simulink model "cic_filter_testing_8"  (Simulink 7.4)
settings: Solver=ode45  StartTime=0.0  StopTime=10000  RelTol=1e-3
undefined symbols (not defined in the file or in its folder): xlRetrieveParam
libraries: xbsIndex_r4 x441
(part 2 of 3)

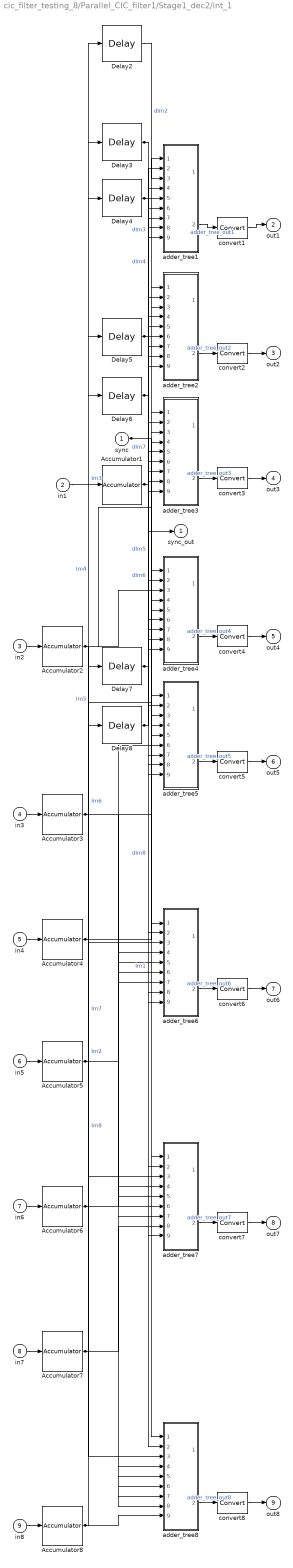
== system cic_filter_testing_8/Parallel_CIC_filter1/Stage1_dec2/int_1 ==
  sync : Inport
  in1 : Inport  Port=2
  in2 : Inport  Port=3
  in3 : Inport  Port=4
  in4 : Inport  Port=5
  in5 : Inport  Port=6
  in6 : Inport  Port=7
  in7 : Inport  Port=8
  in8 : Inport  Port=9
  Accumulator{1..8} (8 alike) : xbsIndex_r4/Accumulator  operation=Add  n_bits=11  overflow=Wrap  scale=1  rst=off  hasbypass=off  en=off  dbl_ovrd=off  use_behavioral_HDL=on  implementation=Fabric  block_type=accum
      settings: block_version=11.4
  Delay{2..8} (7 alike) : xbsIndex_r4/Delay  en=off  latency=1  dbl_ovrd=off  reg_retiming=off  block_type=delay
      settings: block_version=11.4
  adder_tree1 : Subsystem
  adder_tree2 : Subsystem
  adder_tree3 : Subsystem
  adder_tree4 : Subsystem
  adder_tree5 : Subsystem
  adder_tree6 : Subsystem
  adder_tree7 : Subsystem
  adder_tree8 : Subsystem
  convert{1..8} (8 alike) : xbsIndex_r4/Convert  arith_type="Signed  (2's comp)"  n_bits=11  bin_pt=7  quantization=Truncate  overflow=Wrap  latency=0  dbl_ovrd=off  pipeline=off  block_type=convert
      settings: block_version=11.4
  sync_out : Outport
  out1 : Outport  Port=2
  out2 : Outport  Port=3
  out3 : Outport  Port=4
  out4 : Outport  Port=5
  out5 : Outport  Port=6
  out6 : Outport  Port=7
  out7 : Outport  Port=8
  out8 : Outport  Port=9
  wires:
  Accumulator2/1 -> adder_tree8/3(din_2), adder_tree7/3(din_2), adder_tree6/3(din_2), adder_tree5/3(din_2), adder_tree4/3(din_2), adder_tree3/3(din_2), adder_tree2/3(din_2), Delay2/1  "Im2"
  Accumulator3/1 -> adder_tree8/4(din_3), adder_tree7/4(din_3), adder_tree6/4(din_3), adder_tree5/4(din_3), adder_tree4/4(din_3), adder_tree3/4(din_3), Delay3/1  "Im3"
  Accumulator4/1 -> adder_tree8/5(din_4), adder_tree7/5(din_4), adder_tree6/5(din_4), adder_tree5/5(din_4), adder_tree4/5(din_4), Delay4/1  "Im4"
  Accumulator5/1 -> adder_tree8/6(din_5), adder_tree7/6(din_5), adder_tree6/6(din_5), adder_tree5/6(din_5), Delay5/1  "Im5"
  Accumulator6/1 -> adder_tree8/7(din_6), adder_tree7/7(din_6), adder_tree6/7(din_6), Delay6/1  "Im6"
  Accumulator7/1 -> adder_tree8/8(din_7), adder_tree7/8(din_7), Delay7/1  "Im7"
  Accumulator8/1 -> adder_tree8/9(din_8), Delay8/1  "Im8"
  sync/1 -> sync_out/1, adder_tree8/1(sync), adder_tree7/1(sync), adder_tree6/1(sync), adder_tree5/1(sync), adder_tree4/1(sync), adder_tree3/1(sync), adder_tree2/1(sync), adder_tree1/1(sync)
  Accumulator1/1 -> adder_tree8/2(din_1), adder_tree7/2(din_1), adder_tree6/2(din_1), adder_tree5/2(din_1), adder_tree4/2(din_1), adder_tree3/2(din_1), adder_tree2/2(din_1), adder_tree1/2(din_1)  "Im1"
  Delay3/1 -> adder_tree2/4(din_3), adder_tree1/4(din_3)  "dIm3"
  Delay4/1 -> adder_tree3/5(din_4), adder_tree2/5(din_4), adder_tree1/5(din_4)  "dIm4"
  Delay5/1 -> adder_tree4/6(din_5), adder_tree3/6(din_5), adder_tree2/6(din_5), adder_tree1/6(din_5)  "dIm5"
  Delay6/1 -> adder_tree5/7(din_6), adder_tree4/7(din_6), adder_tree3/7(din_6), adder_tree2/7(din_6), adder_tree1/7(din_6)  "dIm6"
  Delay7/1 -> adder_tree6/8(din_7), adder_tree5/8(din_7), adder_tree4/8(din_7), adder_tree3/8(din_7), adder_tree2/8(din_7), adder_tree1/8(din_7)  "dIm7"
  Delay8/1 -> adder_tree7/9(din_8), adder_tree6/9(din_8), adder_tree5/9(din_8), adder_tree4/9(din_8), adder_tree3/9(din_8), adder_tree2/9(din_8), adder_tree1/9(din_8)  "dIm8"
  convert8/1 -> out8/1
  adder_tree8/2(dout) -> convert8/1  "adder_tree_out8"
  convert7/1 -> out7/1
  adder_tree7/2(dout) -> convert7/1  "adder_tree_out7"
  convert6/1 -> out6/1
  adder_tree6/2(dout) -> convert6/1  "adder_tree_out6"
  convert5/1 -> out5/1
  adder_tree5/2(dout) -> convert5/1  "adder_tree_out5"
  convert4/1 -> out4/1
  adder_tree4/2(dout) -> convert4/1  "adder_tree_out4"
  convert3/1 -> out3/1
  adder_tree3/2(dout) -> convert3/1  "adder_tree_out3"
  convert2/1 -> out2/1
  adder_tree2/2(dout) -> convert2/1  "adder_tree_out2"
  convert1/1 -> out1/1
  adder_tree1/2(dout) -> convert1/1  "adder_tree_out1"
  Delay2/1 -> adder_tree1/3(din_2)  "dIm2"
  in8/1 -> Accumulator8/1
  in7/1 -> Accumulator7/1
  in6/1 -> Accumulator6/1
  in5/1 -> Accumulator5/1
  in4/1 -> Accumulator4/1
  in3/1 -> Accumulator3/1
  in2/1 -> Accumulator2/1
  in1/1 -> Accumulator1/1

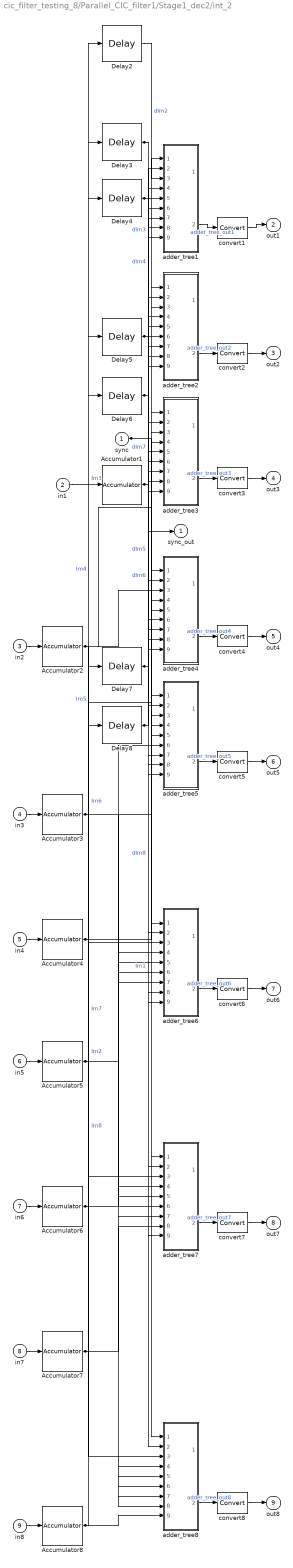
== system cic_filter_testing_8/Parallel_CIC_filter1/Stage1_dec2/int_2 ==
  sync : Inport
  in1 : Inport  Port=2
  in2 : Inport  Port=3
  in3 : Inport  Port=4
  in4 : Inport  Port=5
  in5 : Inport  Port=6
  in6 : Inport  Port=7
  in7 : Inport  Port=8
  in8 : Inport  Port=9
  Accumulator{1..8} (8 alike) : xbsIndex_r4/Accumulator  operation=Add  n_bits=11  overflow=Wrap  scale=1  rst=off  hasbypass=off  en=off  dbl_ovrd=off  use_behavioral_HDL=on  implementation=Fabric  block_type=accum
      settings: block_version=11.4
  Delay{2..8} (7 alike) : xbsIndex_r4/Delay  en=off  latency=1  dbl_ovrd=off  reg_retiming=off  block_type=delay
      settings: block_version=11.4
  adder_tree1 : Subsystem
  adder_tree2 : Subsystem
  adder_tree3 : Subsystem
  adder_tree4 : Subsystem
  adder_tree5 : Subsystem
  adder_tree6 : Subsystem
  adder_tree7 : Subsystem
  adder_tree8 : Subsystem
  convert{1..8} (8 alike) : xbsIndex_r4/Convert  arith_type="Signed  (2's comp)"  n_bits=11  bin_pt=7  quantization=Truncate  overflow=Wrap  latency=0  dbl_ovrd=off  pipeline=off  block_type=convert
      settings: block_version=11.4
  sync_out : Outport
  out1 : Outport  Port=2
  out2 : Outport  Port=3
  out3 : Outport  Port=4
  out4 : Outport  Port=5
  out5 : Outport  Port=6
  out6 : Outport  Port=7
  out7 : Outport  Port=8
  out8 : Outport  Port=9
  wires:
  Accumulator2/1 -> adder_tree8/3(din_2), adder_tree7/3(din_2), adder_tree6/3(din_2), adder_tree5/3(din_2), adder_tree4/3(din_2), adder_tree3/3(din_2), adder_tree2/3(din_2), Delay2/1  "Im2"
  Accumulator3/1 -> adder_tree8/4(din_3), adder_tree7/4(din_3), adder_tree6/4(din_3), adder_tree5/4(din_3), adder_tree4/4(din_3), adder_tree3/4(din_3), Delay3/1  "Im3"
  Accumulator4/1 -> adder_tree8/5(din_4), adder_tree7/5(din_4), adder_tree6/5(din_4), adder_tree5/5(din_4), adder_tree4/5(din_4), Delay4/1  "Im4"
  Accumulator5/1 -> adder_tree8/6(din_5), adder_tree7/6(din_5), adder_tree6/6(din_5), adder_tree5/6(din_5), Delay5/1  "Im5"
  Accumulator6/1 -> adder_tree8/7(din_6), adder_tree7/7(din_6), adder_tree6/7(din_6), Delay6/1  "Im6"
  Accumulator7/1 -> adder_tree8/8(din_7), adder_tree7/8(din_7), Delay7/1  "Im7"
  Accumulator8/1 -> adder_tree8/9(din_8), Delay8/1  "Im8"
  sync/1 -> sync_out/1, adder_tree8/1(sync), adder_tree7/1(sync), adder_tree6/1(sync), adder_tree5/1(sync), adder_tree4/1(sync), adder_tree3/1(sync), adder_tree2/1(sync), adder_tree1/1(sync)
  Accumulator1/1 -> adder_tree8/2(din_1), adder_tree7/2(din_1), adder_tree6/2(din_1), adder_tree5/2(din_1), adder_tree4/2(din_1), adder_tree3/2(din_1), adder_tree2/2(din_1), adder_tree1/2(din_1)  "Im1"
  Delay3/1 -> adder_tree2/4(din_3), adder_tree1/4(din_3)  "dIm3"
  Delay4/1 -> adder_tree3/5(din_4), adder_tree2/5(din_4), adder_tree1/5(din_4)  "dIm4"
  Delay5/1 -> adder_tree4/6(din_5), adder_tree3/6(din_5), adder_tree2/6(din_5), adder_tree1/6(din_5)  "dIm5"
  Delay6/1 -> adder_tree5/7(din_6), adder_tree4/7(din_6), adder_tree3/7(din_6), adder_tree2/7(din_6), adder_tree1/7(din_6)  "dIm6"
  Delay7/1 -> adder_tree6/8(din_7), adder_tree5/8(din_7), adder_tree4/8(din_7), adder_tree3/8(din_7), adder_tree2/8(din_7), adder_tree1/8(din_7)  "dIm7"
  Delay8/1 -> adder_tree7/9(din_8), adder_tree6/9(din_8), adder_tree5/9(din_8), adder_tree4/9(din_8), adder_tree3/9(din_8), adder_tree2/9(din_8), adder_tree1/9(din_8)  "dIm8"
  convert8/1 -> out8/1
  adder_tree8/2(dout) -> convert8/1  "adder_tree_out8"
  convert7/1 -> out7/1
  adder_tree7/2(dout) -> convert7/1  "adder_tree_out7"
  convert6/1 -> out6/1
  adder_tree6/2(dout) -> convert6/1  "adder_tree_out6"
  convert5/1 -> out5/1
  adder_tree5/2(dout) -> convert5/1  "adder_tree_out5"
  convert4/1 -> out4/1
  adder_tree4/2(dout) -> convert4/1  "adder_tree_out4"
  convert3/1 -> out3/1
  adder_tree3/2(dout) -> convert3/1  "adder_tree_out3"
  convert2/1 -> out2/1
  adder_tree2/2(dout) -> convert2/1  "adder_tree_out2"
  convert1/1 -> out1/1
  adder_tree1/2(dout) -> convert1/1  "adder_tree_out1"
  Delay2/1 -> adder_tree1/3(din_2)  "dIm2"
  in8/1 -> Accumulator8/1
  in7/1 -> Accumulator7/1
  in6/1 -> Accumulator6/1
  in5/1 -> Accumulator5/1
  in4/1 -> Accumulator4/1
  in3/1 -> Accumulator3/1
  in2/1 -> Accumulator2/1
  in1/1 -> Accumulator1/1

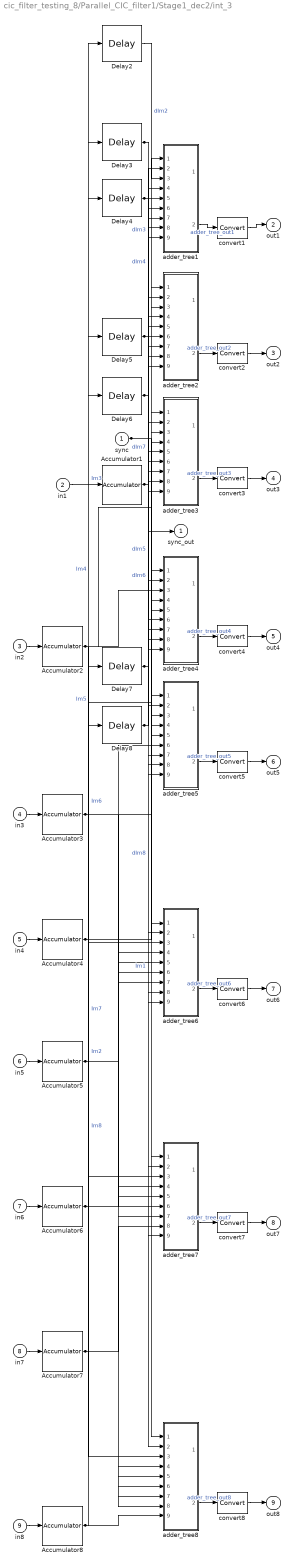
== system cic_filter_testing_8/Parallel_CIC_filter1/Stage1_dec2/int_3 ==
  sync : Inport
  in1 : Inport  Port=2
  in2 : Inport  Port=3
  in3 : Inport  Port=4
  in4 : Inport  Port=5
  in5 : Inport  Port=6
  in6 : Inport  Port=7
  in7 : Inport  Port=8
  in8 : Inport  Port=9
  Accumulator{1..8} (8 alike) : xbsIndex_r4/Accumulator  operation=Add  n_bits=11  overflow=Wrap  scale=1  rst=off  hasbypass=off  en=off  dbl_ovrd=off  use_behavioral_HDL=on  implementation=Fabric  block_type=accum
      settings: block_version=11.4
  Delay{2..8} (7 alike) : xbsIndex_r4/Delay  en=off  latency=1  dbl_ovrd=off  reg_retiming=off  block_type=delay
      settings: block_version=11.4
  adder_tree1 : Subsystem
  adder_tree2 : Subsystem
  adder_tree3 : Subsystem
  adder_tree4 : Subsystem
  adder_tree5 : Subsystem
  adder_tree6 : Subsystem
  adder_tree7 : Subsystem
  adder_tree8 : Subsystem
  convert{1..8} (8 alike) : xbsIndex_r4/Convert  arith_type="Signed  (2's comp)"  n_bits=11  bin_pt=7  quantization=Truncate  overflow=Wrap  latency=0  dbl_ovrd=off  pipeline=off  block_type=convert
      settings: block_version=11.4
  sync_out : Outport
  out1 : Outport  Port=2
  out2 : Outport  Port=3
  out3 : Outport  Port=4
  out4 : Outport  Port=5
  out5 : Outport  Port=6
  out6 : Outport  Port=7
  out7 : Outport  Port=8
  out8 : Outport  Port=9
  wires:
  Accumulator2/1 -> adder_tree8/3(din_2), adder_tree7/3(din_2), adder_tree6/3(din_2), adder_tree5/3(din_2), adder_tree4/3(din_2), adder_tree3/3(din_2), adder_tree2/3(din_2), Delay2/1  "Im2"
  Accumulator3/1 -> adder_tree8/4(din_3), adder_tree7/4(din_3), adder_tree6/4(din_3), adder_tree5/4(din_3), adder_tree4/4(din_3), adder_tree3/4(din_3), Delay3/1  "Im3"
  Accumulator4/1 -> adder_tree8/5(din_4), adder_tree7/5(din_4), adder_tree6/5(din_4), adder_tree5/5(din_4), adder_tree4/5(din_4), Delay4/1  "Im4"
  Accumulator5/1 -> adder_tree8/6(din_5), adder_tree7/6(din_5), adder_tree6/6(din_5), adder_tree5/6(din_5), Delay5/1  "Im5"
  Accumulator6/1 -> adder_tree8/7(din_6), adder_tree7/7(din_6), adder_tree6/7(din_6), Delay6/1  "Im6"
  Accumulator7/1 -> adder_tree8/8(din_7), adder_tree7/8(din_7), Delay7/1  "Im7"
  Accumulator8/1 -> adder_tree8/9(din_8), Delay8/1  "Im8"
  sync/1 -> sync_out/1, adder_tree8/1(sync), adder_tree7/1(sync), adder_tree6/1(sync), adder_tree5/1(sync), adder_tree4/1(sync), adder_tree3/1(sync), adder_tree2/1(sync), adder_tree1/1(sync)
  Accumulator1/1 -> adder_tree8/2(din_1), adder_tree7/2(din_1), adder_tree6/2(din_1), adder_tree5/2(din_1), adder_tree4/2(din_1), adder_tree3/2(din_1), adder_tree2/2(din_1), adder_tree1/2(din_1)  "Im1"
  Delay3/1 -> adder_tree2/4(din_3), adder_tree1/4(din_3)  "dIm3"
  Delay4/1 -> adder_tree3/5(din_4), adder_tree2/5(din_4), adder_tree1/5(din_4)  "dIm4"
  Delay5/1 -> adder_tree4/6(din_5), adder_tree3/6(din_5), adder_tree2/6(din_5), adder_tree1/6(din_5)  "dIm5"
  Delay6/1 -> adder_tree5/7(din_6), adder_tree4/7(din_6), adder_tree3/7(din_6), adder_tree2/7(din_6), adder_tree1/7(din_6)  "dIm6"
  Delay7/1 -> adder_tree6/8(din_7), adder_tree5/8(din_7), adder_tree4/8(din_7), adder_tree3/8(din_7), adder_tree2/8(din_7), adder_tree1/8(din_7)  "dIm7"
  Delay8/1 -> adder_tree7/9(din_8), adder_tree6/9(din_8), adder_tree5/9(din_8), adder_tree4/9(din_8), adder_tree3/9(din_8), adder_tree2/9(din_8), adder_tree1/9(din_8)  "dIm8"
  convert8/1 -> out8/1
  adder_tree8/2(dout) -> convert8/1  "adder_tree_out8"
  convert7/1 -> out7/1
  adder_tree7/2(dout) -> convert7/1  "adder_tree_out7"
  convert6/1 -> out6/1
  adder_tree6/2(dout) -> convert6/1  "adder_tree_out6"
  convert5/1 -> out5/1
  adder_tree5/2(dout) -> convert5/1  "adder_tree_out5"
  convert4/1 -> out4/1
  adder_tree4/2(dout) -> convert4/1  "adder_tree_out4"
  convert3/1 -> out3/1
  adder_tree3/2(dout) -> convert3/1  "adder_tree_out3"
  convert2/1 -> out2/1
  adder_tree2/2(dout) -> convert2/1  "adder_tree_out2"
  convert1/1 -> out1/1
  adder_tree1/2(dout) -> convert1/1  "adder_tree_out1"
  Delay2/1 -> adder_tree1/3(din_2)  "dIm2"
  in8/1 -> Accumulator8/1
  in7/1 -> Accumulator7/1
  in6/1 -> Accumulator6/1
  in5/1 -> Accumulator5/1
  in4/1 -> Accumulator4/1
  in3/1 -> Accumulator3/1
  in2/1 -> Accumulator2/1
  in1/1 -> Accumulator1/1

== system cic_filter_testing_8/Parallel_CIC_filter1/Stage2_dec2/comb_1 ==
  sync_in : Inport
  in1 : Inport  Port=2
  in2 : Inport  Port=3
  Delay2 : xbsIndex_r4/Delay  en=off  latency=1  dbl_ovrd=off  reg_retiming=off  block_type=delay
      settings: block_version=11.4
  sub_blk1 : xbsIndex_r4/AddSub  mode=Subtraction  use_carryin=off  use_carryout=off  en=off  latency=1  precision=User Defined  arith_type="Signed  (2's comp)"  n_bits=14  bin_pt=7  quantization=Truncate  overflow=Wrap  dbl_ovrd=off  use_behavioral_HDL=on  hw_selection=Fabric  pipelined=off  block_type=addsub
  sub_blk2 : xbsIndex_r4/AddSub  mode=Subtraction  use_carryin=off  use_carryout=off  en=off  latency=1  precision=User Defined  arith_type="Signed  (2's comp)"  n_bits=14  bin_pt=7  quantization=Truncate  overflow=Wrap  dbl_ovrd=off  use_behavioral_HDL=on  hw_selection=Fabric  pipelined=off  block_type=addsub
  sync_delay : xbsIndex_r4/Delay  en=off  latency=1  dbl_ovrd=off  reg_retiming=off  block_type=delay
      settings: block_version=11.4
  sync_out : Outport
  out1 : Outport  Port=2
  out2 : Outport  Port=3
  wires:
  in2/1 -> sub_blk2/1, Delay2/1
  in1/1 -> sub_blk2/2, sub_blk1/1
  sync_delay/1 -> sync_out/1
  sync_in/1 -> sync_delay/1
  sub_blk2/1 -> out2/1
  sub_blk1/1 -> out1/1
  Delay2/1 -> sub_blk1/2  "d_in2"

== system cic_filter_testing_8/Parallel_CIC_filter1/Stage2_dec2/comb_2 ==
  sync_in : Inport
  in1 : Inport  Port=2
  in2 : Inport  Port=3
  Delay2 : xbsIndex_r4/Delay  en=off  latency=1  dbl_ovrd=off  reg_retiming=off  block_type=delay
      settings: block_version=11.4
  sub_blk1 : xbsIndex_r4/AddSub  mode=Subtraction  use_carryin=off  use_carryout=off  en=off  latency=1  precision=User Defined  arith_type="Signed  (2's comp)"  n_bits=14  bin_pt=7  quantization=Truncate  overflow=Wrap  dbl_ovrd=off  use_behavioral_HDL=on  hw_selection=Fabric  pipelined=off  block_type=addsub
  sub_blk2 : xbsIndex_r4/AddSub  mode=Subtraction  use_carryin=off  use_carryout=off  en=off  latency=1  precision=User Defined  arith_type="Signed  (2's comp)"  n_bits=14  bin_pt=7  quantization=Truncate  overflow=Wrap  dbl_ovrd=off  use_behavioral_HDL=on  hw_selection=Fabric  pipelined=off  block_type=addsub
  sync_delay : xbsIndex_r4/Delay  en=off  latency=1  dbl_ovrd=off  reg_retiming=off  block_type=delay
      settings: block_version=11.4
  sync_out : Outport
  out1 : Outport  Port=2
  out2 : Outport  Port=3
  wires:
  in2/1 -> sub_blk2/1, Delay2/1
  in1/1 -> sub_blk2/2, sub_blk1/1
  sync_delay/1 -> sync_out/1
  sync_in/1 -> sync_delay/1
  sub_blk2/1 -> out2/1
  sub_blk1/1 -> out1/1
  Delay2/1 -> sub_blk1/2  "d_in2"

== system cic_filter_testing_8/Parallel_CIC_filter1/Stage2_dec2/comb_3 ==
  sync_in : Inport
  in1 : Inport  Port=2
  in2 : Inport  Port=3
  Delay2 : xbsIndex_r4/Delay  en=off  latency=1  dbl_ovrd=off  reg_retiming=off  block_type=delay
      settings: block_version=11.4
  sub_blk1 : xbsIndex_r4/AddSub  mode=Subtraction  use_carryin=off  use_carryout=off  en=off  latency=1  precision=User Defined  arith_type="Signed  (2's comp)"  n_bits=14  bin_pt=7  quantization=Truncate  overflow=Wrap  dbl_ovrd=off  use_behavioral_HDL=on  hw_selection=Fabric  pipelined=off  block_type=addsub
  sub_blk2 : xbsIndex_r4/AddSub  mode=Subtraction  use_carryin=off  use_carryout=off  en=off  latency=1  precision=User Defined  arith_type="Signed  (2's comp)"  n_bits=14  bin_pt=7  quantization=Truncate  overflow=Wrap  dbl_ovrd=off  use_behavioral_HDL=on  hw_selection=Fabric  pipelined=off  block_type=addsub
  sync_delay : xbsIndex_r4/Delay  en=off  latency=1  dbl_ovrd=off  reg_retiming=off  block_type=delay
      settings: block_version=11.4
  sync_out : Outport
  out1 : Outport  Port=2
  out2 : Outport  Port=3
  wires:
  in2/1 -> sub_blk2/1, Delay2/1
  in1/1 -> sub_blk2/2, sub_blk1/1
  sync_delay/1 -> sync_out/1
  sync_in/1 -> sync_delay/1
  sub_blk2/1 -> out2/1
  sub_blk1/1 -> out1/1
  Delay2/1 -> sub_blk1/2  "d_in2"

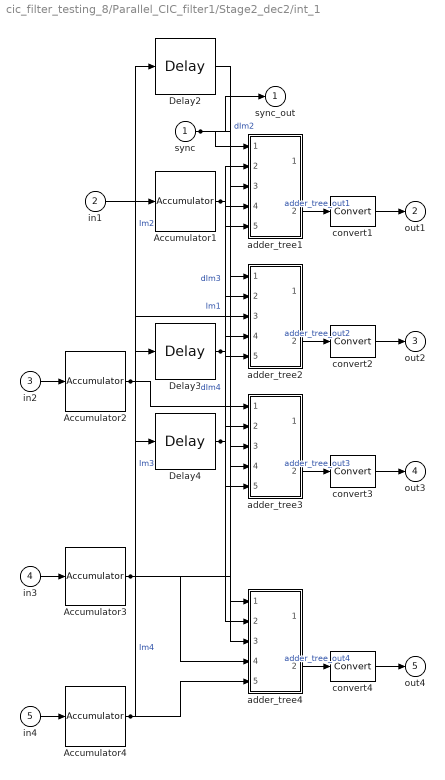
== system cic_filter_testing_8/Parallel_CIC_filter1/Stage2_dec2/int_1 ==
  sync : Inport
  in1 : Inport  Port=2
  in2 : Inport  Port=3
  in3 : Inport  Port=4
  in4 : Inport  Port=5
  Accumulator{1..4} (4 alike) : xbsIndex_r4/Accumulator  operation=Add  n_bits=14  overflow=Wrap  scale=1  rst=off  hasbypass=off  en=off  dbl_ovrd=off  use_behavioral_HDL=on  implementation=Fabric  block_type=accum
      settings: block_version=11.4
  Delay2 : xbsIndex_r4/Delay  en=off  latency=1  dbl_ovrd=off  reg_retiming=off  block_type=delay
      settings: block_version=11.4
  Delay3 : xbsIndex_r4/Delay  en=off  latency=1  dbl_ovrd=off  reg_retiming=off  block_type=delay
      settings: block_version=11.4
  Delay4 : xbsIndex_r4/Delay  en=off  latency=1  dbl_ovrd=off  reg_retiming=off  block_type=delay
      settings: block_version=11.4
  adder_tree1 : Subsystem
  adder_tree2 : Subsystem
  adder_tree3 : Subsystem
  adder_tree4 : Subsystem
  convert{1..4} (4 alike) : xbsIndex_r4/Convert  arith_type="Signed  (2's comp)"  n_bits=14  bin_pt=7  quantization=Truncate  overflow=Wrap  latency=0  dbl_ovrd=off  pipeline=off  block_type=convert
      settings: block_version=11.4
  sync_out : Outport
  out1 : Outport  Port=2
  out2 : Outport  Port=3
  out3 : Outport  Port=4
  out4 : Outport  Port=5
  wires:
  Accumulator2/1 -> adder_tree4/3(din_2), adder_tree3/3(din_2), adder_tree2/3(din_2), Delay2/1  "Im2"
  Accumulator3/1 -> adder_tree4/4(din_3), adder_tree3/4(din_3), Delay3/1  "Im3"
  Accumulator4/1 -> adder_tree4/5(din_4), Delay4/1  "Im4"
  sync/1 -> sync_out/1, adder_tree4/1(sync), adder_tree3/1(sync), adder_tree2/1(sync), adder_tree1/1(sync)
  Accumulator1/1 -> adder_tree4/2(din_1), adder_tree3/2(din_1), adder_tree2/2(din_1), adder_tree1/2(din_1)  "Im1"
  Delay3/1 -> adder_tree2/4(din_3), adder_tree1/4(din_3)  "dIm3"
  Delay4/1 -> adder_tree3/5(din_4), adder_tree2/5(din_4), adder_tree1/5(din_4)  "dIm4"
  convert4/1 -> out4/1
  adder_tree4/2(dout) -> convert4/1  "adder_tree_out4"
  convert3/1 -> out3/1
  adder_tree3/2(dout) -> convert3/1  "adder_tree_out3"
  convert2/1 -> out2/1
  adder_tree2/2(dout) -> convert2/1  "adder_tree_out2"
  convert1/1 -> out1/1
  adder_tree1/2(dout) -> convert1/1  "adder_tree_out1"
  Delay2/1 -> adder_tree1/3(din_2)  "dIm2"
  in4/1 -> Accumulator4/1
  in3/1 -> Accumulator3/1
  in2/1 -> Accumulator2/1
  in1/1 -> Accumulator1/1

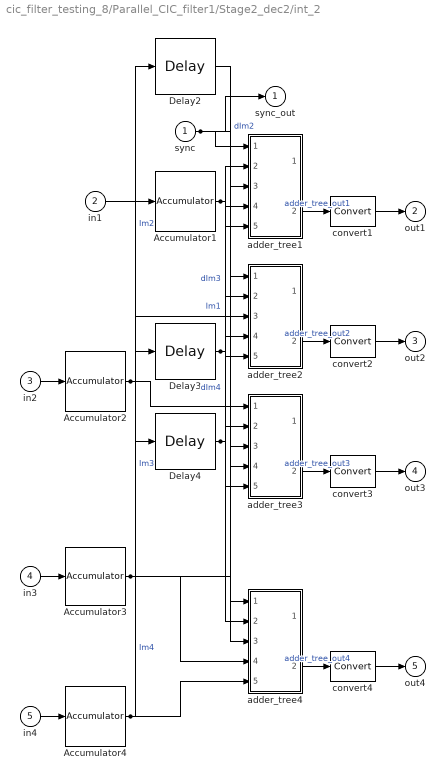
== system cic_filter_testing_8/Parallel_CIC_filter1/Stage2_dec2/int_2 ==
  sync : Inport
  in1 : Inport  Port=2
  in2 : Inport  Port=3
  in3 : Inport  Port=4
  in4 : Inport  Port=5
  Accumulator{1..4} (4 alike) : xbsIndex_r4/Accumulator  operation=Add  n_bits=14  overflow=Wrap  scale=1  rst=off  hasbypass=off  en=off  dbl_ovrd=off  use_behavioral_HDL=on  implementation=Fabric  block_type=accum
      settings: block_version=11.4
  Delay2 : xbsIndex_r4/Delay  en=off  latency=1  dbl_ovrd=off  reg_retiming=off  block_type=delay
      settings: block_version=11.4
  Delay3 : xbsIndex_r4/Delay  en=off  latency=1  dbl_ovrd=off  reg_retiming=off  block_type=delay
      settings: block_version=11.4
  Delay4 : xbsIndex_r4/Delay  en=off  latency=1  dbl_ovrd=off  reg_retiming=off  block_type=delay
      settings: block_version=11.4
  adder_tree1 : Subsystem
  adder_tree2 : Subsystem
  adder_tree3 : Subsystem
  adder_tree4 : Subsystem
  convert{1..4} (4 alike) : xbsIndex_r4/Convert  arith_type="Signed  (2's comp)"  n_bits=14  bin_pt=7  quantization=Truncate  overflow=Wrap  latency=0  dbl_ovrd=off  pipeline=off  block_type=convert
      settings: block_version=11.4
  sync_out : Outport
  out1 : Outport  Port=2
  out2 : Outport  Port=3
  out3 : Outport  Port=4
  out4 : Outport  Port=5
  wires:
  Accumulator2/1 -> adder_tree4/3(din_2), adder_tree3/3(din_2), adder_tree2/3(din_2), Delay2/1  "Im2"
  Accumulator3/1 -> adder_tree4/4(din_3), adder_tree3/4(din_3), Delay3/1  "Im3"
  Accumulator4/1 -> adder_tree4/5(din_4), Delay4/1  "Im4"
  sync/1 -> sync_out/1, adder_tree4/1(sync), adder_tree3/1(sync), adder_tree2/1(sync), adder_tree1/1(sync)
  Accumulator1/1 -> adder_tree4/2(din_1), adder_tree3/2(din_1), adder_tree2/2(din_1), adder_tree1/2(din_1)  "Im1"
  Delay3/1 -> adder_tree2/4(din_3), adder_tree1/4(din_3)  "dIm3"
  Delay4/1 -> adder_tree3/5(din_4), adder_tree2/5(din_4), adder_tree1/5(din_4)  "dIm4"
  convert4/1 -> out4/1
  adder_tree4/2(dout) -> convert4/1  "adder_tree_out4"
  convert3/1 -> out3/1
  adder_tree3/2(dout) -> convert3/1  "adder_tree_out3"
  convert2/1 -> out2/1
  adder_tree2/2(dout) -> convert2/1  "adder_tree_out2"
  convert1/1 -> out1/1
  adder_tree1/2(dout) -> convert1/1  "adder_tree_out1"
  Delay2/1 -> adder_tree1/3(din_2)  "dIm2"
  in4/1 -> Accumulator4/1
  in3/1 -> Accumulator3/1
  in2/1 -> Accumulator2/1
  in1/1 -> Accumulator1/1

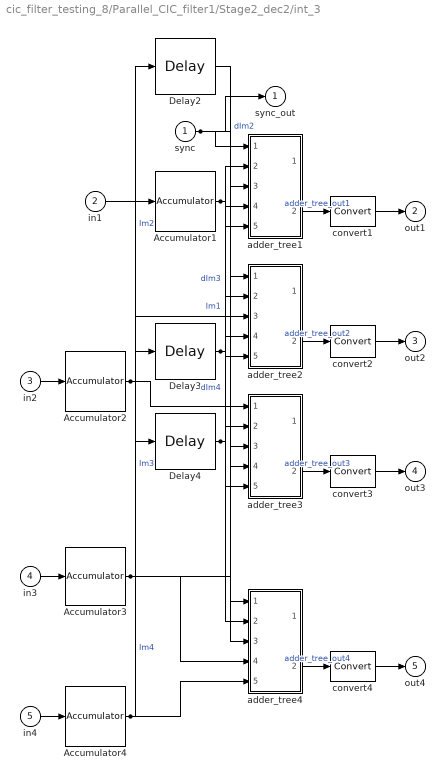
== system cic_filter_testing_8/Parallel_CIC_filter1/Stage2_dec2/int_3 ==
  sync : Inport
  in1 : Inport  Port=2
  in2 : Inport  Port=3
  in3 : Inport  Port=4
  in4 : Inport  Port=5
  Accumulator{1..4} (4 alike) : xbsIndex_r4/Accumulator  operation=Add  n_bits=14  overflow=Wrap  scale=1  rst=off  hasbypass=off  en=off  dbl_ovrd=off  use_behavioral_HDL=on  implementation=Fabric  block_type=accum
      settings: block_version=11.4
  Delay2 : xbsIndex_r4/Delay  en=off  latency=1  dbl_ovrd=off  reg_retiming=off  block_type=delay
      settings: block_version=11.4
  Delay3 : xbsIndex_r4/Delay  en=off  latency=1  dbl_ovrd=off  reg_retiming=off  block_type=delay
      settings: block_version=11.4
  Delay4 : xbsIndex_r4/Delay  en=off  latency=1  dbl_ovrd=off  reg_retiming=off  block_type=delay
      settings: block_version=11.4
  adder_tree1 : Subsystem
  adder_tree2 : Subsystem
  adder_tree3 : Subsystem
  adder_tree4 : Subsystem
  convert{1..4} (4 alike) : xbsIndex_r4/Convert  arith_type="Signed  (2's comp)"  n_bits=14  bin_pt=7  quantization=Truncate  overflow=Wrap  latency=0  dbl_ovrd=off  pipeline=off  block_type=convert
      settings: block_version=11.4
  sync_out : Outport
  out1 : Outport  Port=2
  out2 : Outport  Port=3
  out3 : Outport  Port=4
  out4 : Outport  Port=5
  wires:
  Accumulator2/1 -> adder_tree4/3(din_2), adder_tree3/3(din_2), adder_tree2/3(din_2), Delay2/1  "Im2"
  Accumulator3/1 -> adder_tree4/4(din_3), adder_tree3/4(din_3), Delay3/1  "Im3"
  Accumulator4/1 -> adder_tree4/5(din_4), Delay4/1  "Im4"
  sync/1 -> sync_out/1, adder_tree4/1(sync), adder_tree3/1(sync), adder_tree2/1(sync), adder_tree1/1(sync)
  Accumulator1/1 -> adder_tree4/2(din_1), adder_tree3/2(din_1), adder_tree2/2(din_1), adder_tree1/2(din_1)  "Im1"
  Delay3/1 -> adder_tree2/4(din_3), adder_tree1/4(din_3)  "dIm3"
  Delay4/1 -> adder_tree3/5(din_4), adder_tree2/5(din_4), adder_tree1/5(din_4)  "dIm4"
  convert4/1 -> out4/1
  adder_tree4/2(dout) -> convert4/1  "adder_tree_out4"
  convert3/1 -> out3/1
  adder_tree3/2(dout) -> convert3/1  "adder_tree_out3"
  convert2/1 -> out2/1
  adder_tree2/2(dout) -> convert2/1  "adder_tree_out2"
  convert1/1 -> out1/1
  adder_tree1/2(dout) -> convert1/1  "adder_tree_out1"
  Delay2/1 -> adder_tree1/3(din_2)  "dIm2"
  in4/1 -> Accumulator4/1
  in3/1 -> Accumulator3/1
  in2/1 -> Accumulator2/1
  in1/1 -> Accumulator1/1

== system cic_filter_testing_8/Parallel_CIC_filter1/Stage3_dec2/comb_1 ==
  sync_in : Inport
  in : Inport  Port=2
  Delay : xbsIndex_r4/Delay  en=off  latency=1  dbl_ovrd=off  reg_retiming=off  block_type=delay
      settings: block_version=11.4
  sub_blk1 : xbsIndex_r4/AddSub  mode=Subtraction  use_carryin=off  use_carryout=off  en=off  latency=1  precision=User Defined  arith_type="Signed  (2's comp)"  n_bits=17  bin_pt=7  quantization=Truncate  overflow=Wrap  dbl_ovrd=off  use_behavioral_HDL=on  hw_selection=Fabric  pipelined=off  block_type=addsub
  sync_delay : xbsIndex_r4/Delay  en=off  latency=1  dbl_ovrd=off  reg_retiming=off  block_type=delay
      settings: block_version=11.4
  sync_out : Outport
  out : Outport  Port=2
  wires:
  in/1 -> sub_blk1/1, Delay/1
  sync_delay/1 -> sync_out/1
  sync_in/1 -> sync_delay/1
  sub_blk1/1 -> out/1  "sub_out"
  Delay/1 -> sub_blk1/2  "d_in"

== system cic_filter_testing_8/Parallel_CIC_filter1/Stage3_dec2/comb_2 ==
  sync_in : Inport
  in : Inport  Port=2
  Delay : xbsIndex_r4/Delay  en=off  latency=1  dbl_ovrd=off  reg_retiming=off  block_type=delay
      settings: block_version=11.4
  sub_blk1 : xbsIndex_r4/AddSub  mode=Subtraction  use_carryin=off  use_carryout=off  en=off  latency=1  precision=User Defined  arith_type="Signed  (2's comp)"  n_bits=17  bin_pt=7  quantization=Truncate  overflow=Wrap  dbl_ovrd=off  use_behavioral_HDL=on  hw_selection=Fabric  pipelined=off  block_type=addsub
  sync_delay : xbsIndex_r4/Delay  en=off  latency=1  dbl_ovrd=off  reg_retiming=off  block_type=delay
      settings: block_version=11.4
  sync_out : Outport
  out : Outport  Port=2
  wires:
  in/1 -> sub_blk1/1, Delay/1
  sync_delay/1 -> sync_out/1
  sync_in/1 -> sync_delay/1
  sub_blk1/1 -> out/1  "sub_out"
  Delay/1 -> sub_blk1/2  "d_in"

== system cic_filter_testing_8/Parallel_CIC_filter1/Stage3_dec2/comb_3 ==
  sync_in : Inport
  in : Inport  Port=2
  Delay : xbsIndex_r4/Delay  en=off  latency=1  dbl_ovrd=off  reg_retiming=off  block_type=delay
      settings: block_version=11.4
  sub_blk1 : xbsIndex_r4/AddSub  mode=Subtraction  use_carryin=off  use_carryout=off  en=off  latency=1  precision=User Defined  arith_type="Signed  (2's comp)"  n_bits=17  bin_pt=7  quantization=Truncate  overflow=Wrap  dbl_ovrd=off  use_behavioral_HDL=on  hw_selection=Fabric  pipelined=off  block_type=addsub
  sync_delay : xbsIndex_r4/Delay  en=off  latency=1  dbl_ovrd=off  reg_retiming=off  block_type=delay
      settings: block_version=11.4
  sync_out : Outport
  out : Outport  Port=2
  wires:
  in/1 -> sub_blk1/1, Delay/1
  sync_delay/1 -> sync_out/1
  sync_in/1 -> sync_delay/1
  sub_blk1/1 -> out/1  "sub_out"
  Delay/1 -> sub_blk1/2  "d_in"

== system cic_filter_testing_8/Parallel_CIC_filter1/Stage3_dec2/int_1 ==
  sync : Inport
  in1 : Inport  Port=2
  in2 : Inport  Port=3
  Accumulator1 : xbsIndex_r4/Accumulator  operation=Add  n_bits=17  overflow=Wrap  scale=1  rst=off  hasbypass=off  en=off  dbl_ovrd=off  use_behavioral_HDL=on  implementation=Fabric  block_type=accum
      settings: block_version=11.4
  Accumulator2 : xbsIndex_r4/Accumulator  operation=Add  n_bits=17  overflow=Wrap  scale=1  rst=off  hasbypass=off  en=off  dbl_ovrd=off  use_behavioral_HDL=on  implementation=Fabric  block_type=accum
      settings: block_version=11.4
  Delay2 : xbsIndex_r4/Delay  en=off  latency=1  dbl_ovrd=off  reg_retiming=off  block_type=delay
      settings: block_version=11.4
  adder_tree1 : Subsystem
  adder_tree2 : Subsystem
  convert1 : xbsIndex_r4/Convert  arith_type="Signed  (2's comp)"  n_bits=17  bin_pt=7  quantization=Truncate  overflow=Wrap  latency=0  dbl_ovrd=off  pipeline=off  block_type=convert
      settings: block_version=11.4
  convert2 : xbsIndex_r4/Convert  arith_type="Signed  (2's comp)"  n_bits=17  bin_pt=7  quantization=Truncate  overflow=Wrap  latency=0  dbl_ovrd=off  pipeline=off  block_type=convert
      settings: block_version=11.4
  sync_out : Outport
  out1 : Outport  Port=2
  out2 : Outport  Port=3
  wires:
  Accumulator2/1 -> adder_tree2/3(din_2), Delay2/1  "Im2"
  sync/1 -> sync_out/1, adder_tree2/1(sync), adder_tree1/1(sync)
  Accumulator1/1 -> adder_tree2/2(din_1), adder_tree1/2(din_1)  "Im1"
  convert2/1 -> out2/1
  adder_tree2/2(dout) -> convert2/1  "adder_tree_out2"
  convert1/1 -> out1/1
  adder_tree1/2(dout) -> convert1/1  "adder_tree_out1"
  Delay2/1 -> adder_tree1/3(din_2)  "dIm2"
  in2/1 -> Accumulator2/1
  in1/1 -> Accumulator1/1

== system cic_filter_testing_8/Parallel_CIC_filter1/Stage3_dec2/int_2 ==
  sync : Inport
  in1 : Inport  Port=2
  in2 : Inport  Port=3
  Accumulator1 : xbsIndex_r4/Accumulator  operation=Add  n_bits=17  overflow=Wrap  scale=1  rst=off  hasbypass=off  en=off  dbl_ovrd=off  use_behavioral_HDL=on  implementation=Fabric  block_type=accum
      settings: block_version=11.4
  Accumulator2 : xbsIndex_r4/Accumulator  operation=Add  n_bits=17  overflow=Wrap  scale=1  rst=off  hasbypass=off  en=off  dbl_ovrd=off  use_behavioral_HDL=on  implementation=Fabric  block_type=accum
      settings: block_version=11.4
  Delay2 : xbsIndex_r4/Delay  en=off  latency=1  dbl_ovrd=off  reg_retiming=off  block_type=delay
      settings: block_version=11.4
  adder_tree1 : Subsystem
  adder_tree2 : Subsystem
  convert1 : xbsIndex_r4/Convert  arith_type="Signed  (2's comp)"  n_bits=17  bin_pt=7  quantization=Truncate  overflow=Wrap  latency=0  dbl_ovrd=off  pipeline=off  block_type=convert
      settings: block_version=11.4
  convert2 : xbsIndex_r4/Convert  arith_type="Signed  (2's comp)"  n_bits=17  bin_pt=7  quantization=Truncate  overflow=Wrap  latency=0  dbl_ovrd=off  pipeline=off  block_type=convert
      settings: block_version=11.4
  sync_out : Outport
  out1 : Outport  Port=2
  out2 : Outport  Port=3
  wires:
  Accumulator2/1 -> adder_tree2/3(din_2), Delay2/1  "Im2"
  sync/1 -> sync_out/1, adder_tree2/1(sync), adder_tree1/1(sync)
  Accumulator1/1 -> adder_tree2/2(din_1), adder_tree1/2(din_1)  "Im1"
  convert2/1 -> out2/1
  adder_tree2/2(dout) -> convert2/1  "adder_tree_out2"
  convert1/1 -> out1/1
  adder_tree1/2(dout) -> convert1/1  "adder_tree_out1"
  Delay2/1 -> adder_tree1/3(din_2)  "dIm2"
  in2/1 -> Accumulator2/1
  in1/1 -> Accumulator1/1

== system cic_filter_testing_8/Parallel_CIC_filter1/Stage3_dec2/int_3 ==
  sync : Inport
  in1 : Inport  Port=2
  in2 : Inport  Port=3
  Accumulator1 : xbsIndex_r4/Accumulator  operation=Add  n_bits=17  overflow=Wrap  scale=1  rst=off  hasbypass=off  en=off  dbl_ovrd=off  use_behavioral_HDL=on  implementation=Fabric  block_type=accum
      settings: block_version=11.4
  Accumulator2 : xbsIndex_r4/Accumulator  operation=Add  n_bits=17  overflow=Wrap  scale=1  rst=off  hasbypass=off  en=off  dbl_ovrd=off  use_behavioral_HDL=on  implementation=Fabric  block_type=accum
      settings: block_version=11.4
  Delay2 : xbsIndex_r4/Delay  en=off  latency=1  dbl_ovrd=off  reg_retiming=off  block_type=delay
      settings: block_version=11.4
  adder_tree1 : Subsystem
  adder_tree2 : Subsystem
  convert1 : xbsIndex_r4/Convert  arith_type="Signed  (2's comp)"  n_bits=17  bin_pt=7  quantization=Truncate  overflow=Wrap  latency=0  dbl_ovrd=off  pipeline=off  block_type=convert
      settings: block_version=11.4
  convert2 : xbsIndex_r4/Convert  arith_type="Signed  (2's comp)"  n_bits=17  bin_pt=7  quantization=Truncate  overflow=Wrap  latency=0  dbl_ovrd=off  pipeline=off  block_type=convert
      settings: block_version=11.4
  sync_out : Outport
  out1 : Outport  Port=2
  out2 : Outport  Port=3
  wires:
  Accumulator2/1 -> adder_tree2/3(din_2), Delay2/1  "Im2"
  sync/1 -> sync_out/1, adder_tree2/1(sync), adder_tree1/1(sync)
  Accumulator1/1 -> adder_tree2/2(din_1), adder_tree1/2(din_1)  "Im1"
  convert2/1 -> out2/1
  adder_tree2/2(dout) -> convert2/1  "adder_tree_out2"
  convert1/1 -> out1/1
  adder_tree1/2(dout) -> convert1/1  "adder_tree_out1"
  Delay2/1 -> adder_tree1/3(din_2)  "dIm2"
  in2/1 -> Accumulator2/1
  in1/1 -> Accumulator1/1

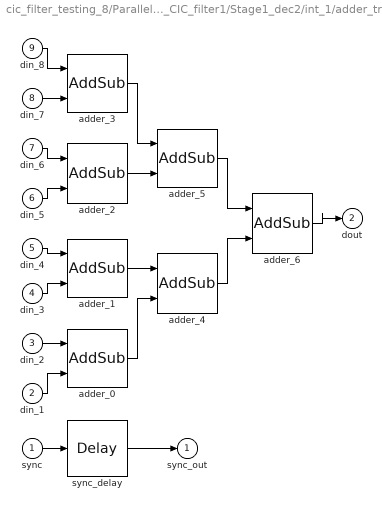
== system cic_filter_testing_8/Parallel_CIC_filter1/Stage1_dec2/int_1/adder_tree1 ==
  sync : Inport
  din_1 : Inport  Port=2
  din_2 : Inport  Port=3
  din_3 : Inport  Port=4
  din_4 : Inport  Port=5
  din_5 : Inport  Port=6
  din_6 : Inport  Port=7
  din_7 : Inport  Port=8
  din_8 : Inport  Port=9
  adder_{0..6} (7 alike) : xbsIndex_r4/AddSub  mode=Addition  use_carryin=off  use_carryout=off  en=off  latency=1  precision=Full  arith_type=Unsigned  n_bits=18  bin_pt=17  quantization="Round  (unbiased: +/- Inf)"  overflow=Wrap  dbl_ovrd=off  use_behavioral_HDL=on  hw_selection=Fabric  pipelined=off  block_type=addsub
  sync_delay : xbsIndex_r4/Delay  en=off  latency=3  dbl_ovrd=off  reg_retiming=off  block_type=delay
      settings: block_version=11.4
  sync_out : Outport
  dout : Outport  Port=2
  wires:
  adder_6/1 -> dout/1
  adder_4/1 -> adder_6/2
  adder_5/1 -> adder_6/1
  adder_2/1 -> adder_5/2
  adder_3/1 -> adder_5/1
  adder_0/1 -> adder_4/2
  adder_1/1 -> adder_4/1
  din_7/1 -> adder_3/2
  din_8/1 -> adder_3/1
  din_5/1 -> adder_2/2
  din_6/1 -> adder_2/1
  din_3/1 -> adder_1/2
  din_4/1 -> adder_1/1
  din_1/1 -> adder_0/2
  din_2/1 -> adder_0/1
  sync_delay/1 -> sync_out/1
  sync/1 -> sync_delay/1

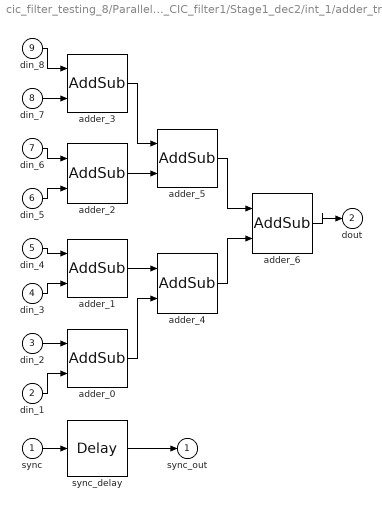
== system cic_filter_testing_8/Parallel_CIC_filter1/Stage1_dec2/int_1/adder_tree2 ==
  sync : Inport
  din_1 : Inport  Port=2
  din_2 : Inport  Port=3
  din_3 : Inport  Port=4
  din_4 : Inport  Port=5
  din_5 : Inport  Port=6
  din_6 : Inport  Port=7
  din_7 : Inport  Port=8
  din_8 : Inport  Port=9
  adder_{0..6} (7 alike) : xbsIndex_r4/AddSub  mode=Addition  use_carryin=off  use_carryout=off  en=off  latency=1  precision=Full  arith_type=Unsigned  n_bits=18  bin_pt=17  quantization="Round  (unbiased: +/- Inf)"  overflow=Wrap  dbl_ovrd=off  use_behavioral_HDL=on  hw_selection=Fabric  pipelined=off  block_type=addsub
  sync_delay : xbsIndex_r4/Delay  en=off  latency=3  dbl_ovrd=off  reg_retiming=off  block_type=delay
      settings: block_version=11.4
  sync_out : Outport
  dout : Outport  Port=2
  wires:
  adder_6/1 -> dout/1
  adder_4/1 -> adder_6/2
  adder_5/1 -> adder_6/1
  adder_2/1 -> adder_5/2
  adder_3/1 -> adder_5/1
  adder_0/1 -> adder_4/2
  adder_1/1 -> adder_4/1
  din_7/1 -> adder_3/2
  din_8/1 -> adder_3/1
  din_5/1 -> adder_2/2
  din_6/1 -> adder_2/1
  din_3/1 -> adder_1/2
  din_4/1 -> adder_1/1
  din_1/1 -> adder_0/2
  din_2/1 -> adder_0/1
  sync_delay/1 -> sync_out/1
  sync/1 -> sync_delay/1

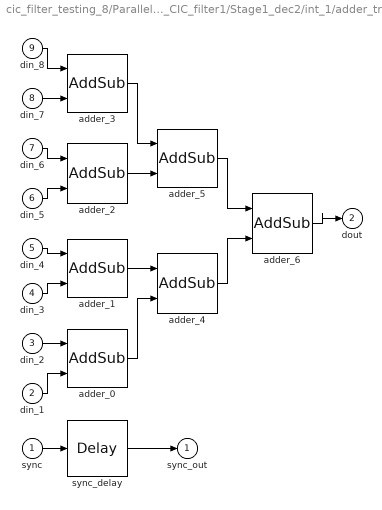
== system cic_filter_testing_8/Parallel_CIC_filter1/Stage1_dec2/int_1/adder_tree3 ==
  sync : Inport
  din_1 : Inport  Port=2
  din_2 : Inport  Port=3
  din_3 : Inport  Port=4
  din_4 : Inport  Port=5
  din_5 : Inport  Port=6
  din_6 : Inport  Port=7
  din_7 : Inport  Port=8
  din_8 : Inport  Port=9
  adder_{0..6} (7 alike) : xbsIndex_r4/AddSub  mode=Addition  use_carryin=off  use_carryout=off  en=off  latency=1  precision=Full  arith_type=Unsigned  n_bits=18  bin_pt=17  quantization="Round  (unbiased: +/- Inf)"  overflow=Wrap  dbl_ovrd=off  use_behavioral_HDL=on  hw_selection=Fabric  pipelined=off  block_type=addsub
  sync_delay : xbsIndex_r4/Delay  en=off  latency=3  dbl_ovrd=off  reg_retiming=off  block_type=delay
      settings: block_version=11.4
  sync_out : Outport
  dout : Outport  Port=2
  wires:
  adder_6/1 -> dout/1
  adder_4/1 -> adder_6/2
  adder_5/1 -> adder_6/1
  adder_2/1 -> adder_5/2
  adder_3/1 -> adder_5/1
  adder_0/1 -> adder_4/2
  adder_1/1 -> adder_4/1
  din_7/1 -> adder_3/2
  din_8/1 -> adder_3/1
  din_5/1 -> adder_2/2
  din_6/1 -> adder_2/1
  din_3/1 -> adder_1/2
  din_4/1 -> adder_1/1
  din_1/1 -> adder_0/2
  din_2/1 -> adder_0/1
  sync_delay/1 -> sync_out/1
  sync/1 -> sync_delay/1

== system cic_filter_testing_8/Parallel_CIC_filter1/Stage1_dec2/int_1/adder_tree4 ==
  sync : Inport
  din_1 : Inport  Port=2
  din_2 : Inport  Port=3
  din_3 : Inport  Port=4
  din_4 : Inport  Port=5
  din_5 : Inport  Port=6
  din_6 : Inport  Port=7
  din_7 : Inport  Port=8
  din_8 : Inport  Port=9
  adder_{0..6} (7 alike) : xbsIndex_r4/AddSub  mode=Addition  use_carryin=off  use_carryout=off  en=off  latency=1  precision=Full  arith_type=Unsigned  n_bits=18  bin_pt=17  quantization="Round  (unbiased: +/- Inf)"  overflow=Wrap  dbl_ovrd=off  use_behavioral_HDL=on  hw_selection=Fabric  pipelined=off  block_type=addsub
  sync_delay : xbsIndex_r4/Delay  en=off  latency=3  dbl_ovrd=off  reg_retiming=off  block_type=delay
      settings: block_version=11.4
  sync_out : Outport
  dout : Outport  Port=2
  wires:
  adder_6/1 -> dout/1
  adder_4/1 -> adder_6/2
  adder_5/1 -> adder_6/1
  adder_2/1 -> adder_5/2
  adder_3/1 -> adder_5/1
  adder_0/1 -> adder_4/2
  adder_1/1 -> adder_4/1
  din_7/1 -> adder_3/2
  din_8/1 -> adder_3/1
  din_5/1 -> adder_2/2
  din_6/1 -> adder_2/1
  din_3/1 -> adder_1/2
  din_4/1 -> adder_1/1
  din_1/1 -> adder_0/2
  din_2/1 -> adder_0/1
  sync_delay/1 -> sync_out/1
  sync/1 -> sync_delay/1

== system cic_filter_testing_8/Parallel_CIC_filter1/Stage1_dec2/int_1/adder_tree5 ==
  sync : Inport
  din_1 : Inport  Port=2
  din_2 : Inport  Port=3
  din_3 : Inport  Port=4
  din_4 : Inport  Port=5
  din_5 : Inport  Port=6
  din_6 : Inport  Port=7
  din_7 : Inport  Port=8
  din_8 : Inport  Port=9
  adder_{0..6} (7 alike) : xbsIndex_r4/AddSub  mode=Addition  use_carryin=off  use_carryout=off  en=off  latency=1  precision=Full  arith_type=Unsigned  n_bits=18  bin_pt=17  quantization="Round  (unbiased: +/- Inf)"  overflow=Wrap  dbl_ovrd=off  use_behavioral_HDL=on  hw_selection=Fabric  pipelined=off  block_type=addsub
  sync_delay : xbsIndex_r4/Delay  en=off  latency=3  dbl_ovrd=off  reg_retiming=off  block_type=delay
      settings: block_version=11.4
  sync_out : Outport
  dout : Outport  Port=2
  wires:
  adder_6/1 -> dout/1
  adder_4/1 -> adder_6/2
  adder_5/1 -> adder_6/1
  adder_2/1 -> adder_5/2
  adder_3/1 -> adder_5/1
  adder_0/1 -> adder_4/2
  adder_1/1 -> adder_4/1
  din_7/1 -> adder_3/2
  din_8/1 -> adder_3/1
  din_5/1 -> adder_2/2
  din_6/1 -> adder_2/1
  din_3/1 -> adder_1/2
  din_4/1 -> adder_1/1
  din_1/1 -> adder_0/2
  din_2/1 -> adder_0/1
  sync_delay/1 -> sync_out/1
  sync/1 -> sync_delay/1

== system cic_filter_testing_8/Parallel_CIC_filter1/Stage1_dec2/int_1/adder_tree6 ==
  sync : Inport
  din_1 : Inport  Port=2
  din_2 : Inport  Port=3
  din_3 : Inport  Port=4
  din_4 : Inport  Port=5
  din_5 : Inport  Port=6
  din_6 : Inport  Port=7
  din_7 : Inport  Port=8
  din_8 : Inport  Port=9
  adder_{0..6} (7 alike) : xbsIndex_r4/AddSub  mode=Addition  use_carryin=off  use_carryout=off  en=off  latency=1  precision=Full  arith_type=Unsigned  n_bits=18  bin_pt=17  quantization="Round  (unbiased: +/- Inf)"  overflow=Wrap  dbl_ovrd=off  use_behavioral_HDL=on  hw_selection=Fabric  pipelined=off  block_type=addsub
  sync_delay : xbsIndex_r4/Delay  en=off  latency=3  dbl_ovrd=off  reg_retiming=off  block_type=delay
      settings: block_version=11.4
  sync_out : Outport
  dout : Outport  Port=2
  wires:
  adder_6/1 -> dout/1
  adder_4/1 -> adder_6/2
  adder_5/1 -> adder_6/1
  adder_2/1 -> adder_5/2
  adder_3/1 -> adder_5/1
  adder_0/1 -> adder_4/2
  adder_1/1 -> adder_4/1
  din_7/1 -> adder_3/2
  din_8/1 -> adder_3/1
  din_5/1 -> adder_2/2
  din_6/1 -> adder_2/1
  din_3/1 -> adder_1/2
  din_4/1 -> adder_1/1
  din_1/1 -> adder_0/2
  din_2/1 -> adder_0/1
  sync_delay/1 -> sync_out/1
  sync/1 -> sync_delay/1

== system cic_filter_testing_8/Parallel_CIC_filter1/Stage1_dec2/int_1/adder_tree7 ==
  sync : Inport
  din_1 : Inport  Port=2
  din_2 : Inport  Port=3
  din_3 : Inport  Port=4
  din_4 : Inport  Port=5
  din_5 : Inport  Port=6
  din_6 : Inport  Port=7
  din_7 : Inport  Port=8
  din_8 : Inport  Port=9
  adder_{0..6} (7 alike) : xbsIndex_r4/AddSub  mode=Addition  use_carryin=off  use_carryout=off  en=off  latency=1  precision=Full  arith_type=Unsigned  n_bits=18  bin_pt=17  quantization="Round  (unbiased: +/- Inf)"  overflow=Wrap  dbl_ovrd=off  use_behavioral_HDL=on  hw_selection=Fabric  pipelined=off  block_type=addsub
  sync_delay : xbsIndex_r4/Delay  en=off  latency=3  dbl_ovrd=off  reg_retiming=off  block_type=delay
      settings: block_version=11.4
  sync_out : Outport
  dout : Outport  Port=2
  wires:
  adder_6/1 -> dout/1
  adder_4/1 -> adder_6/2
  adder_5/1 -> adder_6/1
  adder_2/1 -> adder_5/2
  adder_3/1 -> adder_5/1
  adder_0/1 -> adder_4/2
  adder_1/1 -> adder_4/1
  din_7/1 -> adder_3/2
  din_8/1 -> adder_3/1
  din_5/1 -> adder_2/2
  din_6/1 -> adder_2/1
  din_3/1 -> adder_1/2
  din_4/1 -> adder_1/1
  din_1/1 -> adder_0/2
  din_2/1 -> adder_0/1
  sync_delay/1 -> sync_out/1
  sync/1 -> sync_delay/1

== system cic_filter_testing_8/Parallel_CIC_filter1/Stage1_dec2/int_1/adder_tree8 ==
  sync : Inport
  din_1 : Inport  Port=2
  din_2 : Inport  Port=3
  din_3 : Inport  Port=4
  din_4 : Inport  Port=5
  din_5 : Inport  Port=6
  din_6 : Inport  Port=7
  din_7 : Inport  Port=8
  din_8 : Inport  Port=9
  adder_{0..6} (7 alike) : xbsIndex_r4/AddSub  mode=Addition  use_carryin=off  use_carryout=off  en=off  latency=1  precision=Full  arith_type=Unsigned  n_bits=18  bin_pt=17  quantization="Round  (unbiased: +/- Inf)"  overflow=Wrap  dbl_ovrd=off  use_behavioral_HDL=on  hw_selection=Fabric  pipelined=off  block_type=addsub
  sync_delay : xbsIndex_r4/Delay  en=off  latency=3  dbl_ovrd=off  reg_retiming=off  block_type=delay
      settings: block_version=11.4
  sync_out : Outport
  dout : Outport  Port=2
  wires:
  adder_6/1 -> dout/1
  adder_4/1 -> adder_6/2
  adder_5/1 -> adder_6/1
  adder_2/1 -> adder_5/2
  adder_3/1 -> adder_5/1
  adder_0/1 -> adder_4/2
  adder_1/1 -> adder_4/1
  din_7/1 -> adder_3/2
  din_8/1 -> adder_3/1
  din_5/1 -> adder_2/2
  din_6/1 -> adder_2/1
  din_3/1 -> adder_1/2
  din_4/1 -> adder_1/1
  din_1/1 -> adder_0/2
  din_2/1 -> adder_0/1
  sync_delay/1 -> sync_out/1
  sync/1 -> sync_delay/1

== system cic_filter_testing_8/Parallel_CIC_filter1/Stage1_dec2/int_2/adder_tree1 ==
  sync : Inport
  din_1 : Inport  Port=2
  din_2 : Inport  Port=3
  din_3 : Inport  Port=4
  din_4 : Inport  Port=5
  din_5 : Inport  Port=6
  din_6 : Inport  Port=7
  din_7 : Inport  Port=8
  din_8 : Inport  Port=9
  adder_{0..6} (7 alike) : xbsIndex_r4/AddSub  mode=Addition  use_carryin=off  use_carryout=off  en=off  latency=1  precision=Full  arith_type=Unsigned  n_bits=18  bin_pt=17  quantization="Round  (unbiased: +/- Inf)"  overflow=Wrap  dbl_ovrd=off  use_behavioral_HDL=on  hw_selection=Fabric  pipelined=off  block_type=addsub
  sync_delay : xbsIndex_r4/Delay  en=off  latency=3  dbl_ovrd=off  reg_retiming=off  block_type=delay
      settings: block_version=11.4
  sync_out : Outport
  dout : Outport  Port=2
  wires:
  adder_6/1 -> dout/1
  adder_4/1 -> adder_6/2
  adder_5/1 -> adder_6/1
  adder_2/1 -> adder_5/2
  adder_3/1 -> adder_5/1
  adder_0/1 -> adder_4/2
  adder_1/1 -> adder_4/1
  din_7/1 -> adder_3/2
  din_8/1 -> adder_3/1
  din_5/1 -> adder_2/2
  din_6/1 -> adder_2/1
  din_3/1 -> adder_1/2
  din_4/1 -> adder_1/1
  din_1/1 -> adder_0/2
  din_2/1 -> adder_0/1
  sync_delay/1 -> sync_out/1
  sync/1 -> sync_delay/1

== system cic_filter_testing_8/Parallel_CIC_filter1/Stage1_dec2/int_2/adder_tree2 ==
  sync : Inport
  din_1 : Inport  Port=2
  din_2 : Inport  Port=3
  din_3 : Inport  Port=4
  din_4 : Inport  Port=5
  din_5 : Inport  Port=6
  din_6 : Inport  Port=7
  din_7 : Inport  Port=8
  din_8 : Inport  Port=9
  adder_{0..6} (7 alike) : xbsIndex_r4/AddSub  mode=Addition  use_carryin=off  use_carryout=off  en=off  latency=1  precision=Full  arith_type=Unsigned  n_bits=18  bin_pt=17  quantization="Round  (unbiased: +/- Inf)"  overflow=Wrap  dbl_ovrd=off  use_behavioral_HDL=on  hw_selection=Fabric  pipelined=off  block_type=addsub
  sync_delay : xbsIndex_r4/Delay  en=off  latency=3  dbl_ovrd=off  reg_retiming=off  block_type=delay
      settings: block_version=11.4
  sync_out : Outport
  dout : Outport  Port=2
  wires:
  adder_6/1 -> dout/1
  adder_4/1 -> adder_6/2
  adder_5/1 -> adder_6/1
  adder_2/1 -> adder_5/2
  adder_3/1 -> adder_5/1
  adder_0/1 -> adder_4/2
  adder_1/1 -> adder_4/1
  din_7/1 -> adder_3/2
  din_8/1 -> adder_3/1
  din_5/1 -> adder_2/2
  din_6/1 -> adder_2/1
  din_3/1 -> adder_1/2
  din_4/1 -> adder_1/1
  din_1/1 -> adder_0/2
  din_2/1 -> adder_0/1
  sync_delay/1 -> sync_out/1
  sync/1 -> sync_delay/1

== system cic_filter_testing_8/Parallel_CIC_filter1/Stage1_dec2/int_2/adder_tree3 ==
  sync : Inport
  din_1 : Inport  Port=2
  din_2 : Inport  Port=3
  din_3 : Inport  Port=4
  din_4 : Inport  Port=5
  din_5 : Inport  Port=6
  din_6 : Inport  Port=7
  din_7 : Inport  Port=8
  din_8 : Inport  Port=9
  adder_{0..6} (7 alike) : xbsIndex_r4/AddSub  mode=Addition  use_carryin=off  use_carryout=off  en=off  latency=1  precision=Full  arith_type=Unsigned  n_bits=18  bin_pt=17  quantization="Round  (unbiased: +/- Inf)"  overflow=Wrap  dbl_ovrd=off  use_behavioral_HDL=on  hw_selection=Fabric  pipelined=off  block_type=addsub
  sync_delay : xbsIndex_r4/Delay  en=off  latency=3  dbl_ovrd=off  reg_retiming=off  block_type=delay
      settings: block_version=11.4
  sync_out : Outport
  dout : Outport  Port=2
  wires:
  adder_6/1 -> dout/1
  adder_4/1 -> adder_6/2
  adder_5/1 -> adder_6/1
  adder_2/1 -> adder_5/2
  adder_3/1 -> adder_5/1
  adder_0/1 -> adder_4/2
  adder_1/1 -> adder_4/1
  din_7/1 -> adder_3/2
  din_8/1 -> adder_3/1
  din_5/1 -> adder_2/2
  din_6/1 -> adder_2/1
  din_3/1 -> adder_1/2
  din_4/1 -> adder_1/1
  din_1/1 -> adder_0/2
  din_2/1 -> adder_0/1
  sync_delay/1 -> sync_out/1
  sync/1 -> sync_delay/1

== system cic_filter_testing_8/Parallel_CIC_filter1/Stage1_dec2/int_2/adder_tree4 ==
  sync : Inport
  din_1 : Inport  Port=2
  din_2 : Inport  Port=3
  din_3 : Inport  Port=4
  din_4 : Inport  Port=5
  din_5 : Inport  Port=6
  din_6 : Inport  Port=7
  din_7 : Inport  Port=8
  din_8 : Inport  Port=9
  adder_{0..6} (7 alike) : xbsIndex_r4/AddSub  mode=Addition  use_carryin=off  use_carryout=off  en=off  latency=1  precision=Full  arith_type=Unsigned  n_bits=18  bin_pt=17  quantization="Round  (unbiased: +/- Inf)"  overflow=Wrap  dbl_ovrd=off  use_behavioral_HDL=on  hw_selection=Fabric  pipelined=off  block_type=addsub
  sync_delay : xbsIndex_r4/Delay  en=off  latency=3  dbl_ovrd=off  reg_retiming=off  block_type=delay
      settings: block_version=11.4
  sync_out : Outport
  dout : Outport  Port=2
  wires:
  adder_6/1 -> dout/1
  adder_4/1 -> adder_6/2
  adder_5/1 -> adder_6/1
  adder_2/1 -> adder_5/2
  adder_3/1 -> adder_5/1
  adder_0/1 -> adder_4/2
  adder_1/1 -> adder_4/1
  din_7/1 -> adder_3/2
  din_8/1 -> adder_3/1
  din_5/1 -> adder_2/2
  din_6/1 -> adder_2/1
  din_3/1 -> adder_1/2
  din_4/1 -> adder_1/1
  din_1/1 -> adder_0/2
  din_2/1 -> adder_0/1
  sync_delay/1 -> sync_out/1
  sync/1 -> sync_delay/1

== system cic_filter_testing_8/Parallel_CIC_filter1/Stage1_dec2/int_2/adder_tree5 ==
  sync : Inport
  din_1 : Inport  Port=2
  din_2 : Inport  Port=3
  din_3 : Inport  Port=4
  din_4 : Inport  Port=5
  din_5 : Inport  Port=6
  din_6 : Inport  Port=7
  din_7 : Inport  Port=8
  din_8 : Inport  Port=9
  adder_{0..6} (7 alike) : xbsIndex_r4/AddSub  mode=Addition  use_carryin=off  use_carryout=off  en=off  latency=1  precision=Full  arith_type=Unsigned  n_bits=18  bin_pt=17  quantization="Round  (unbiased: +/- Inf)"  overflow=Wrap  dbl_ovrd=off  use_behavioral_HDL=on  hw_selection=Fabric  pipelined=off  block_type=addsub
  sync_delay : xbsIndex_r4/Delay  en=off  latency=3  dbl_ovrd=off  reg_retiming=off  block_type=delay
      settings: block_version=11.4
  sync_out : Outport
  dout : Outport  Port=2
  wires:
  adder_6/1 -> dout/1
  adder_4/1 -> adder_6/2
  adder_5/1 -> adder_6/1
  adder_2/1 -> adder_5/2
  adder_3/1 -> adder_5/1
  adder_0/1 -> adder_4/2
  adder_1/1 -> adder_4/1
  din_7/1 -> adder_3/2
  din_8/1 -> adder_3/1
  din_5/1 -> adder_2/2
  din_6/1 -> adder_2/1
  din_3/1 -> adder_1/2
  din_4/1 -> adder_1/1
  din_1/1 -> adder_0/2
  din_2/1 -> adder_0/1
  sync_delay/1 -> sync_out/1
  sync/1 -> sync_delay/1

== system cic_filter_testing_8/Parallel_CIC_filter1/Stage1_dec2/int_2/adder_tree6 ==
  sync : Inport
  din_1 : Inport  Port=2
  din_2 : Inport  Port=3
  din_3 : Inport  Port=4
  din_4 : Inport  Port=5
  din_5 : Inport  Port=6
  din_6 : Inport  Port=7
  din_7 : Inport  Port=8
  din_8 : Inport  Port=9
  adder_{0..6} (7 alike) : xbsIndex_r4/AddSub  mode=Addition  use_carryin=off  use_carryout=off  en=off  latency=1  precision=Full  arith_type=Unsigned  n_bits=18  bin_pt=17  quantization="Round  (unbiased: +/- Inf)"  overflow=Wrap  dbl_ovrd=off  use_behavioral_HDL=on  hw_selection=Fabric  pipelined=off  block_type=addsub
  sync_delay : xbsIndex_r4/Delay  en=off  latency=3  dbl_ovrd=off  reg_retiming=off  block_type=delay
      settings: block_version=11.4
  sync_out : Outport
  dout : Outport  Port=2
  wires:
  adder_6/1 -> dout/1
  adder_4/1 -> adder_6/2
  adder_5/1 -> adder_6/1
  adder_2/1 -> adder_5/2
  adder_3/1 -> adder_5/1
  adder_0/1 -> adder_4/2
  adder_1/1 -> adder_4/1
  din_7/1 -> adder_3/2
  din_8/1 -> adder_3/1
  din_5/1 -> adder_2/2
  din_6/1 -> adder_2/1
  din_3/1 -> adder_1/2
  din_4/1 -> adder_1/1
  din_1/1 -> adder_0/2
  din_2/1 -> adder_0/1
  sync_delay/1 -> sync_out/1
  sync/1 -> sync_delay/1
